simulink model "TEORICO_Respueste_en_tiempo"  (Simulink 10.2)
settings: Solver=ode45  StartTime=0.0  StopTime=3  RelTol=1e-6  EnableMultiTasking=on
values from neighbouring files (symbols this model uses):
  a = 4.1    [TEORICO_Respuesta_en_frecuencia.m]
  c = 3.1    [TEORICO_Respuesta_en_frecuencia.m]
  k = 102    [TEORICO_Respuesta_en_frecuencia.m]
  Kd = 2.1899    [TEORICO_Respuesta_en_frecuencia.m]
  Kdc = 0.1242    [TEORICO_Respuesta_en_frecuencia.m]
  Ki = 0    [TEORICO_Respuesta_en_frecuencia.m]
  Kic = 0    [TEORICO_Respuesta_en_frecuencia.m]
  Kp = 8.8105    [TEORICO_Respuesta_en_frecuencia.m]
  Kpc = 4.405    [TEORICO_Respuesta_en_frecuencia.m]
libraries: simulink_need_slupdate x2
settings Model: Creator=Rober  LastModifiedBy=diego
settings DataIOCC: LimitDataPoints=on
settings OptimizationCC: ExpressionDepthLimit=2147483647  InitFltsAndDblsToZero=on
settings DebuggingCC: SaveWithParameterizedLinksMsg=none  SignalResolutionControl=TryResolveAllWithWarning  SolverPrmCheckMsg=warning  MultiTaskDSMMsg=warning  MultiTaskCondExecSysMsg=none  StateNameClashWarn=warning
settings GRTTargetCC: TargetFcnLib=ansi_tfl_tmw.mat
settings ConfigComp: CovSFcnEnable=off

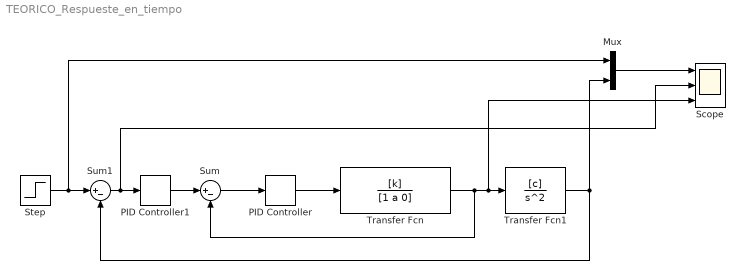
== system TEORICO_Respueste_en_tiempo ==
  Mux : Mux  Inputs=2
  PID Controller : simulink_need_slupdate/PID Controller  P=Kpc  I=Kic  D=Kdc
  PID Controller1 : simulink_need_slupdate/PID Controller  P=Kp  I=Ki  D=Kd
  Scope : Scope  NumInputPorts=3
  Step : Step  Time=0  SampleTime=0
  Sum : Sum  Inputs=|+-
  Sum1 : Sum  Inputs=|+-
  Transfer Fcn : TransferFcn  Numerator=[k]  Denominator=[1 a 0]
  Transfer Fcn1 : TransferFcn  Numerator=[c]  Denominator=[1 0 0]
  wires:
  Transfer Fcn/1 -> Scope/3, Transfer Fcn1/1, Sum/2
  PID Controller/1 -> Transfer Fcn/1
  Sum/1 -> PID Controller/1
  PID Controller1/1 -> Sum/1
  Transfer Fcn1/1 -> Mux/2, Sum1/2
  Sum1/1 -> Scope/2, PID Controller1/1
  Step/1 -> Mux/1, Sum1/1
  Mux/1 -> Scope/1
